simulink model "Segway_simulink_model"  (R2018a)
settings: Solver=VariableStepAuto  StartTime=0.0  StopTime=20  RelTol=1e-3
values from neighbouring files (symbols this model uses):
  A = [0,                  0,            1,                          0 ... (first row only)    [Run_me_first.m]
  Ad = sys_d.a    [Run_me_first.m]
  B = [0 ; 0 ; 1/(mw) ; 1/(L*mw)]    [Run_me_first.m]
  Bd = sys_d.b    [Run_me_first.m]
  Cd = sys_d.c    [Run_me_first.m]
  d1 = 0.01    [Run_me_first.m]
  d2 = 0.01    [Run_me_first.m]
  g = 9.8    [Run_me_first.m]
  k_lqr = lqr(A,B,Q1,R1)    [Run_me_first.m]
  L = 1    [Run_me_first.m]
  mp = 1    [Run_me_first.m]
  mw = 2    [Run_me_first.m]
  Ts = 0.1    [Run_me_first.m]
  x0 = [0 ; 5*pi/180 ; 0 ; 0]    [Run_me_first.m]
undefined symbols (not defined in the file or in its folder): k_d, Ob
settings Model: Creator=Hamas Saeed  LastModifiedBy=Hamas Saeed

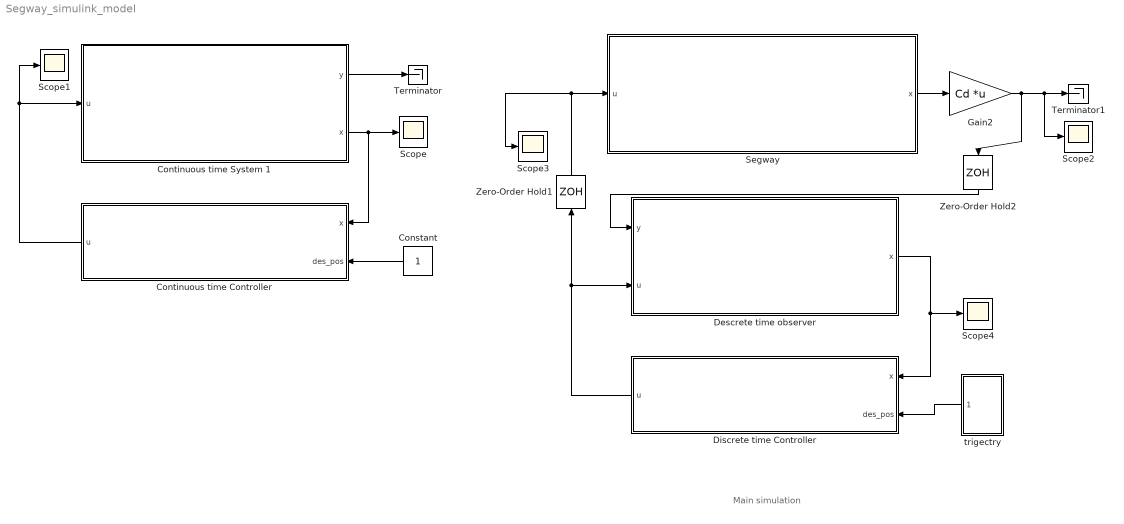
== system Segway_simulink_model ==
  note: Main simulation
  " Descrete time observer " : Subsystem
  Constant : Constant
  Continuous time Controller : Subsystem
  Continuous time System 1 : Subsystem
  Discrete time Controller : Subsystem
  Gain2 : Gain  Gain=Cd  Multiplication=Matrix(K*u)
  Scope{,1..4} (5 alike) : Scope
  "Segway " : Subsystem
  Terminator : Terminator
  Terminator1 : Terminator
  Zero-Order Hold1 : ZeroOrderHold  SampleTime=Ts
  Zero-Order Hold2 : ZeroOrderHold  SampleTime=Ts
  trigectry : Subsystem
  wires:
  Continuous time System 1/1(y) -> Terminator/1
  Continuous time System 1/2(x) -> Continuous time Controller/1(x), Scope/1
  Continuous time Controller/1(u) -> Scope1/1, Continuous time System 1/1(u)
  Constant/1 -> Continuous time Controller/2(des_pos)
  Discrete time Controller/1(u) -> Zero-Order Hold1/1, " Descrete time observer "/2(u)
  Zero-Order Hold1/1 -> Scope3/1, "Segway "/1(u)
  " Descrete time observer "/1(x) -> Discrete time Controller/1(x), Scope4/1
  "Segway "/1(x) -> Gain2/1
  Gain2/1 -> Zero-Order Hold2/1, Scope2/1, Terminator1/1
  trigectry/1(pos_ref) -> Discrete time Controller/2(des_pos)
  Zero-Order Hold2/1 -> " Descrete time observer "/1(y)

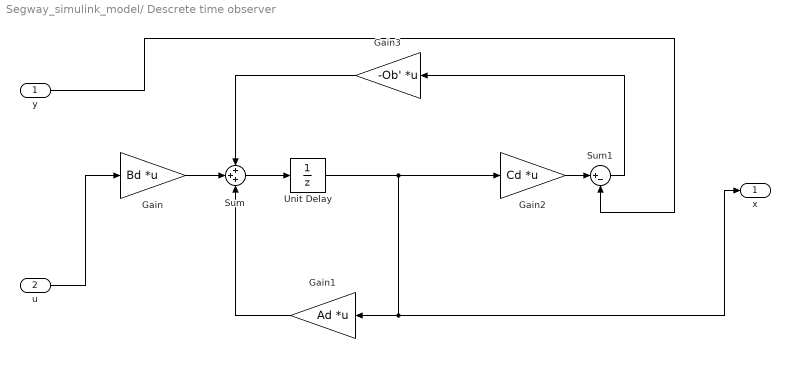
== system Segway_simulink_model/ Descrete time observer  ==
  y : Inport
  u : Inport  Port=2
  Gain : Gain  Gain=Bd  Multiplication=Matrix(K*u)
  Gain1 : Gain  Gain=Ad  Multiplication=Matrix(K*u)
  Gain2 : Gain  Gain=Cd  Multiplication=Matrix(K*u)
  Gain3 : Gain  Gain=-Ob'  Multiplication=Matrix(K*u)
  Sum : Sum  Inputs=+++
  Sum1 : Sum  Inputs=|+-
  Unit Delay : UnitDelay  InitialCondition=x0*0  SampleTime=-1
  x : Outport
  wires:
  Gain2/1 -> Sum1/1
  Unit Delay/1 -> Gain1/1, x/1, Gain2/1
  Sum/1 -> Unit Delay/1
  u/1 -> Gain/1
  y/1 -> Sum1/2
  Gain/1 -> Sum/2
  Gain3/1 -> Sum/1
  Gain1/1 -> Sum/3
  Sum1/1 -> Gain3/1

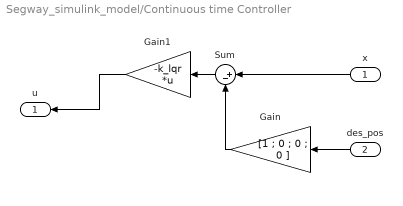
== system Segway_simulink_model/Continuous time Controller ==
  x : Inport
  des_pos : Inport  Port=2
  Gain : Gain  Gain=[1 ; 0 ; 0 ; 0 ]
  Gain1 : Gain  Gain=-k_lqr  Multiplication=Matrix(K*u)
  Sum : Sum  Inputs=|+-
  u : Outport
  wires:
  Gain1/1 -> u/1
  des_pos/1 -> Gain/1
  Sum/1 -> Gain1/1
  x/1 -> Sum/1
  Gain/1 -> Sum/2

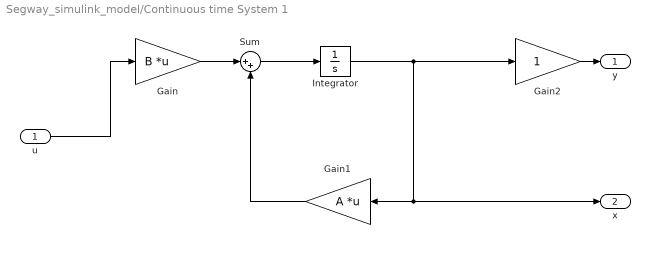
== system Segway_simulink_model/Continuous time System 1 ==
  u : Inport
  Gain : Gain  Gain=B  Multiplication=Matrix(K*u)
  Gain1 : Gain  Gain=A  Multiplication=Matrix(K*u)
  Gain2 : Gain
  Integrator : Integrator  InitialCondition=x0
  Sum : Sum  Inputs=|++
  y : Outport
  x : Outport  Port=2
  wires:
  Gain2/1 -> y/1
  Integrator/1 -> x/1, Gain1/1, Gain2/1
  Gain/1 -> Sum/1
  Sum/1 -> Integrator/1
  u/1 -> Gain/1
  Gain1/1 -> Sum/2

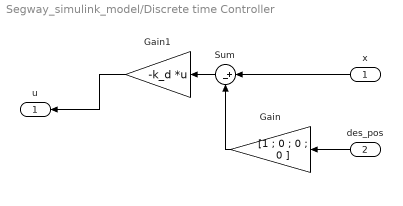
== system Segway_simulink_model/Discrete time Controller ==
  x : Inport
  des_pos : Inport  Port=2
  Gain : Gain  Gain=[1 ; 0 ; 0 ; 0 ]
  Gain1 : Gain  Gain=-k_d  Multiplication=Matrix(K*u)
  Sum : Sum  Inputs=|+-
  u : Outport
  wires:
  Gain1/1 -> u/1
  des_pos/1 -> Gain/1
  Sum/1 -> Gain1/1
  x/1 -> Sum/1
  Gain/1 -> Sum/2

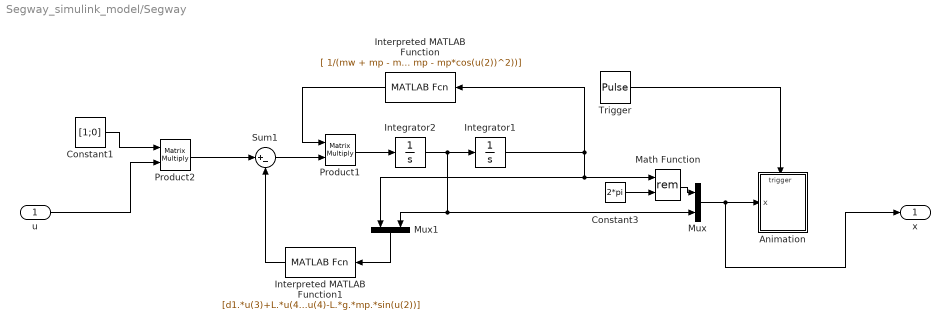
== system Segway_simulink_model/Segway  ==
  u : Inport
  Animation : Subsystem
  Constant1 : Constant  Value=[1;0]
  Constant3 : Constant  Value=2*pi
  Integrator1 : Integrator  InitialCondition=x0(1:2)
  Integrator2 : Integrator  InitialCondition=x0(3:4)
  Interpreted MATLAB Function : MATLABFcn  MATLABFcn="[ 1/(mw + mp - mp*cos(u(2))^2),        cos(u(2))/(L*(mw + mp - mp*cos(u(2))^2)); cos(u(2))/(L*(mw + mp - mp*cos(u(2))^2)), (mw + mp)/(L^2*mp*(mw + mp - mp*cos(u(2))^2))]"  Output1D=off
  Interpreted MATLAB Function1 : MATLABFcn  MATLABFcn=[d1.*u(3)+L.*u(4).^2.*mp.*sin(u(2));d2.*u(4)-L.*g.*mp.*sin(u(2))]
  Math Function : Math  Operator=rem  SaturateOnIntegerOverflow=on
  Mux : Mux  Inputs=2
  Mux1 : Mux  Inputs=2
  Product1 : Product  Multiplication=Matrix(*)
  Product2 : Product  Multiplication=Matrix(*)
  Sum1 : Sum  Inputs=|+-
  Trigger : DiscretePulseGenerator  PulseType=Time based  Period=0.1  PulseWidth=50
  x : Outport
  wires:
  Integrator2/1 -> Mux/2, Mux1/2, Integrator1/1
  u/1 -> Product2/2
  Constant1/1 -> Product2/1
  Math Function/1 -> Mux/1
  Interpreted MATLAB Function1/1 -> Sum1/2
  Constant3/1 -> Math Function/2
  Sum1/1 -> Product1/2
  Mux/1 -> Animation/1(x), x/1
  Product2/1 -> Sum1/1
  Product1/1 -> Integrator2/1
  Interpreted MATLAB Function/1 -> Product1/1
  Trigger/1 -> Animation/Trigger
  Mux1/1 -> Interpreted MATLAB Function1/1
  Integrator1/1 -> Interpreted MATLAB Function/1, Mux1/1, Math Function/1

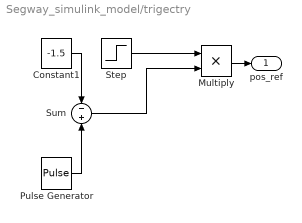
== system Segway_simulink_model/trigectry ==
  Constant1 : Constant  Value=-1.5
  Multiply : Product
  Pulse Generator : DiscretePulseGenerator  PulseType=Time based  Period=5  PulseWidth=25
  Step : Step  Time=5  SampleTime=0
  Sum : Sum  Inputs=-|+
  pos_ref : Outport
  wires:
  Pulse Generator/1 -> Sum/2
  Sum/1 -> Multiply/2
  Constant1/1 -> Sum/1
  Multiply/1 -> pos_ref/1
  Step/1 -> Multiply/1

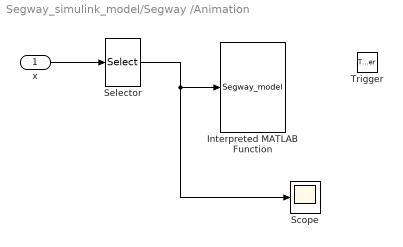
== system Segway_simulink_model/Segway /Animation ==
  x : Inport
  Trigger : TriggerPort  VariantControl=(inherit)  PortDimensions=1
  Interpreted MATLAB Function : MATLABFcn  MATLABFcn=Segway_model  OutputDimensions=0
  Scope : Scope
  Selector : Selector  InputPortWidth=4  IndexOptions=Index vector (dialog)  Indices=[1:2]  OutputSizes=1
  wires:
  x/1 -> Selector/1
  Selector/1 -> Scope/1, Interpreted MATLAB Function/1
